simulink model "SLemba_CPG_startup"  (R2024a)
settings: Solver=ode113  StartTime=0.0  StopTime=10  MaxStep=1e-3  RelTol=1e-5  AbsTol=1e-5
InitFcn:
  | parameters;
  | initBusObjects;
  | loadCPGParam_startup;
values from neighbouring files (symbols this model uses):
  kx_sol = out.kx(1)    [loadCPGParam_startup.m]
  tst_sol = out.tst(1)    [loadCPGParam_startup.m]
  tsw_sol = out.tsw(1)    [loadCPGParam_startup.m]
  y_sol = out.q(2,1)    [loadCPGParam_startup.m]
undefined symbols (not defined in the file or in its folder): Init
settings Model: Creator=heath  LastModifiedBy=Mechatronics
settings SolverCC: ZeroCrossControl=EnableAll
settings DebuggingCC: AlgebraicLoopMsg=none

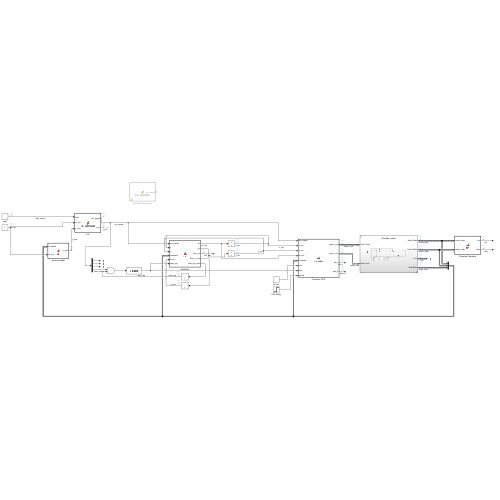
[thumbnail: Simulink's stored preview of the top-level diagram]
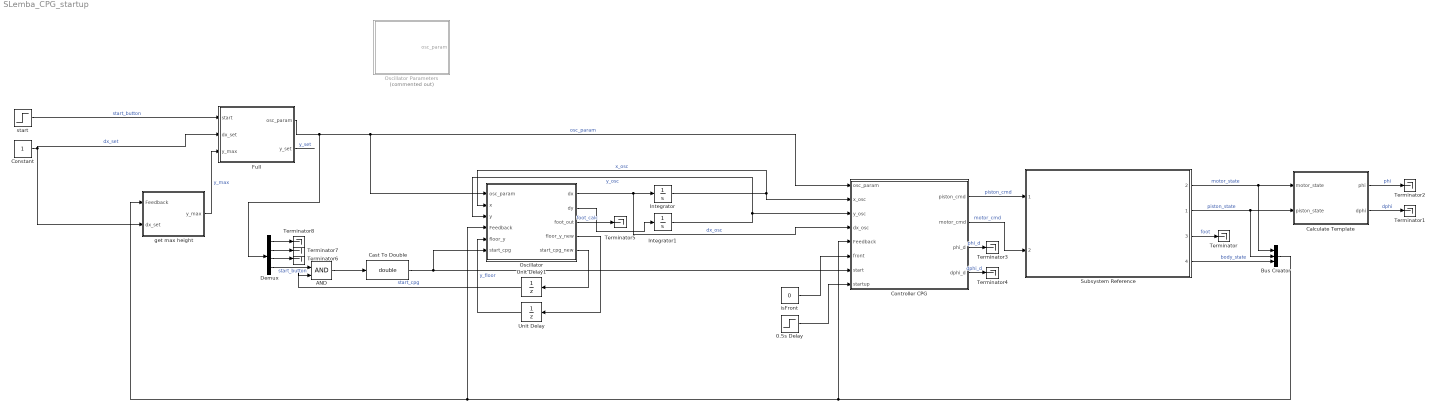
== system SLemba_CPG_startup ==
  0.5s Delay : Step  Time=0.001  SampleTime=0
  AND : Logic  IconShape=distinctive  AllPortsSameDT=off  OutDataTypeStr=boolean
  Bus Creator : BusCreator  Inputs=3  OutDataTypeStr=Bus: State
      settings: InheritFromInputs=off
  Calculate Template : MATLAB Function  TreatAsAtomicUnit=on
  Cast To Double : DataTypeConversion  OutDataTypeStr=double  SaturateOnIntegerOverflow=off  RndMeth=Floor
  Constant : Constant
  Controller CPG : MATLAB Function  TreatAsAtomicUnit=on
  Demux : Demux
  Full : MATLAB Function  TreatAsAtomicUnit=on
  Integrator : Integrator  InitialCondition=Init.CPG(1)
  Integrator1 : Integrator  InitialCondition=Init.CPG(2)
  Oscillator : MATLAB Function  TreatAsAtomicUnit=on
  Oscillator Parameters : MATLAB Function  Commented=on  TreatAsAtomicUnit=on
  Subsystem Reference : Subsystem  ReferencedSubsystem=SLemba_model
      settings: PortSchema="{\"entries\":[{\"content\":{\"sides\":[{\"content\":{\"connectorIds\":[\"In1\",\"In2\"]},\"type\":\"ConnectorPlacement.EquallySpacedRectSide\",\"uuid\":\"d72a35c2-6749-4eaa-8584-fa64d0dc3e1c\"},{\"content\":{\"connectorIds\":[\"Out2\",\"Out1\",\"Out3\",\"Out4\"],\"side\":\"RIGHT\"},\"type\":\"ConnectorPlacement.EquallySpacedRectSide\",\"uuid\":\"d76b7912-ed10-4044-b6e4-c8872f57f584\"},{\"content\":{\"side\":\"TOP\"},\"type\":\"ConnectorPlacement.EquallySpacedRectSide\",\"uuid\":\"b81d1af6-43ba-45da-aadf-2679a7ef4974\"}]},\"type\":\"ConnectorPlacement.EquallySpacedConnector\",\"uuid\":\"64dd74d6-47ac-4ba4-b7a1-dc32513bde35\"}],\"packageUris\":[\"http://schema.mathworks.com/mf0/Connector/R2020b\"],\"version\":\"1.0\"}"
  Terminator{,1..8} (9 alike) : Terminator
  Unit Delay : UnitDelay  SampleTime=-1  HasFrameUpgradeWarning=on
  Unit Delay1 : UnitDelay  SampleTime=-1  HasFrameUpgradeWarning=on
  get max height : MATLAB Function  TreatAsAtomicUnit=on
  isFront : Constant  Value=0
  start : Step  Time=0.002  SampleTime=0
  wires:
  isFront/1 -> Controller CPG/6(front)
  Controller CPG/1(piston_cmd) -> Subsystem Reference/1  "piston_cmd"
  Controller CPG/2(motor_cmd) -> Subsystem Reference/2  "motor_cmd"
  Subsystem Reference/3 -> Terminator/1  "foot"
  Controller CPG/3(phi_d) -> Terminator3/1  "phi_d"
  Controller CPG/4(dphi_d) -> Terminator4/1  "dphi_d"
  Calculate Template/1(phi) -> Terminator2/1  "phi"
  Calculate Template/2(dphi) -> Terminator1/1  "dphi"
  Oscillator/1(dx) -> Controller CPG/4(dx_osc), Integrator/1  "dx_osc"
  Oscillator/2(dy) -> Integrator1/1
  Oscillator/4(floor_y_new) -> Unit Delay/1
  Unit Delay/1 -> Oscillator/5(floor_y)  "y_floor"
  Oscillator/3(foot_out) -> Terminator5/1  "foot_calc"
  start/1 -> Full/1(start)  "start_button"
  Oscillator/5(start_cpg_new) -> Unit Delay1/1
  Subsystem Reference/2 -> Bus Creator/1, Calculate Template/1(motor_state)  "motor_state"
  Subsystem Reference/1 -> Calculate Template/2(piston_state), Bus Creator/2  "piston_state"
  Subsystem Reference/4 -> Bus Creator/3  "body_state"
  Bus Creator/1 -> Controller CPG/5(Feedback), get max height/1(Feedback), Oscillator/4(Feedback)
  0.5s Delay/1 -> Controller CPG/8(startup)
  Constant/1 -> get max height/2(dx_set), Full/2(dx_set)  "dx_set"
  Full/1(osc_param) -> Demux/1, Oscillator/1(osc_param), Controller CPG/1(osc_param)  "osc_param"
  Unit Delay1/1 -> AND/2  "start_cpg"
  Demux/1 -> Terminator8/1
  Demux/2 -> Terminator7/1
  Demux/3 -> Terminator6/1
  Demux/4 -> AND/1  "start_button"
  AND/1 -> Cast To Double/1
  Cast To Double/1 -> Controller CPG/7(start), Oscillator/6(start_cpg)
  get max height/1(y_max) -> Full/3(y_max)  "y_max"
  Full/2(y_set) -> ?  "y_set"
  Integrator/1 -> Controller CPG/2(x_osc), Oscillator/2(x)  "x_osc"
  Integrator1/1 -> Oscillator/3(y), Controller CPG/3(y_osc)  "y_osc"

== matlab function SLemba_CPG_startup/Controller CPG ==
  settings: updateMethod=DISCRETE
  data: osc_param input; x_osc input; piston_cmd output Bus: PistonCmd; y_osc input; dx_osc input; Feedback input Bus: State; front input; start input; startup input double; motor_cmd output Bus: MotorCmd; phi_d output; dphi_d output
function [piston_cmd,motor_cmd,phi_d,dphi_d] = Controller(osc_param, x_osc,y_osc,dx_osc,Feedback,front, start, startup)

persistent state_control % 1 = wait, 2 = startup, 3 = stop

if isempty(state_control)
    state_control = 1;
end


motor_state = Feedback.Motor; piston_state = Feedback.Piston;

kx = osc_param(3);

l = piston_state.p;
dl = piston_state.v;
th = motor_state.q;

if (front)
    direction = -1;
else
    direction = 1;
end

% set command
phi_d = direction*x_osc*kx + pi/2;
dphi_d = direction*dx_osc*kx;
if (y_osc>0) 
    if(x_osc>0)
        ue = 0; ur = 1;
    else
            ue = 1; ur = 1;
    end
else
    ue = 1; ur = 0;
end

kp = 250;
kd = 10;

% % Testing
% % ----------
% ue = 1; ur = 0;
% phi_d = pi/2; dphi_d = 0;
% kp = 250;kd = 5;
% % ---------

if start == 0
    ue = 0; ur = 1;
    phi_d = pi/2; dphi_d = 0;
end

switch(state_control)
    case 1
        if startup == 1
            state_control = 2;
        end
end

switch(state_control)
    case 2
        piston_cmd.ue = ue;
        piston_cmd.ur = ur;
        
        motor_cmd.q = th_calc(phi_d,l);
        motor_cmd.w = dth_calc(phi_calc(th,l),l,dphi_d,dl);
        motor_cmd.Kp = kp;
        motor_cmd.Kd = kd;
        motor_cmd.tff = 0;
    otherwise
        piston_cmd.ue = 0;
        piston_cmd.ur = 0;
        
        motor_cmd.q = 0;
        motor_cmd.w = 0;
        motor_cmd.Kp = 0;
        motor_cmd.Kd = 0;
        motor_cmd.tff = 0;
end

== matlab function SLemba_CPG_startup/Oscillator ==
  settings: updateMethod=DISCRETE
  data: osc_param input; x input size=1; dx output size=1; y input; Feedback input; dy output; foot_out output; floor_y_new output; floor_y input; start_cpg input; start_cpg_new output
function [dx,dy,foot_out,floor_y_new,start_cpg_new] = CPG(osc_param,x,y,Feedback, floor_y, start_cpg)%,dy_lift, fit)%dq_osc = CPG(input_osc)%
% x = input_osc.x_osc; y = input_osc.y_osc; osc_param = input_osc.osc_param;
% Body_state = input_osc.Body_state; Piston_state = input_osc.Piston_state; Motor_state = input_osc.Motor_state;

persistent thrown

if isempty(thrown)
    thrown = 0;
end

Body_state = Feedback.Body; Motor_state = Feedback.Motor; Piston_state = Feedback.Piston;

x_body = Body_state.x; y_body = Body_state.y;
dx_body = Body_state.dx; dy_body = Body_state.dy;
th = Motor_state.q; dth = Motor_state.w;
l = Piston_state.p; dl = Piston_state.v;

thk = thk_calc(th,l); tha = tha_calc(th,l);
dthk = dthk_calc(th,l,dth,dl); dtha = dtha_calc(th,l,dth,dl);

foot = foot_Func(x_body,y_body,th,l,thk,tha,dx_body,dy_body,dth,dl,dthk,dtha);

y_foot = foot(2);
dy_foot = foot(4);

% update floor height based on accelerometer impact
% only activates if system is running and osc is in correct quadrant
ddy_tol = 30;
if (Body_state.ddy > ddy_tol && osc_param(4) && x<-0.5)
    floor_y = y_foot;
end

% start cpg if in correct state once thrown
dy_tol = 0.2;

if dy_body>dy_tol && osc_param(4)
    thrown = 1;
end

if(thrown && dy_body<0)
% if(osc_param(4))
    start_cpg_new = 1;
else
    start_cpg_new = start_cpg;
end

y_foot = y_foot - floor_y;

foot(2) = y_foot;
foot_out = foot;

floor_y_new = floor_y;

tst = osc_param(1);
tsw = osc_param(2);

% constants
mu = 1;
F_1 = 50;
gamma = 10;
b = 100;


% if(dy_lift>0)
%     coeff = fit.coeff;
% 
%     tsw_new = coeff(1) + coeff(2)*tst + coeff(3)*dy_lift + coeff(4)*tst^2 + coeff(5)*tst*dy_lift + coeff(6)*dy_lift^2;
%     if (tsw_new>tst)
%         tsw = tsw_new;
%     end
% end


T = tst + tsw;
d = tsw/T;
% 
% % 3 frequencies with quadrant crossover
% omega_1 = pi/(T*d);
% omega_2 = omega_1;
% omega_3 = pi/(T - T*d);

k = 1; % 2 for extension at half way
e = 0;%0.4;

% 3 frequencies with quadrant crossover
omega_1 = (pi*k - 2*d*e + 2*d*e*k + pi)/(2*T*d*k);
omega_2 = k*omega_1;
omega_3 = (pi*k - 2*d*e + 2*d*e*k + pi)/(T - T*d + T*k - T*d*k);

% polar coordinates
r = sqrt(x^2 + y^2);
th = atan2(y,x);
% th = atan(y/x);
% if (x <= 0)
%     th = pi + atan(y/x);
% end

% 3 frequencies with quadrant cross over
k1 = omega_1/((exp(-b*(x))+1)*(exp(-b*y)+1));
k2 = omega_2/((exp(b*(x))+1)*(exp(-b*y)+1));
k3 = omega_3/(exp(b*y)+1);
omega = k1 + k2 + k3;

f = @(v) 1 + 0.5*cos(v)*tanh(sin(2*v));
f_dash = @(v) cos(v)*cos(2*v)*(sech(sin(2*v)))^2-0.5*sin(v)*tanh(sin(2*v));

% oscillation
dth = omega;
dr = mu*omega*f_dash(th) + gamma*(mu*f(th)-r);

% change in x
dx = dr*cos(th) - r*sin(th)*dth;

if (y_foot <= 0 && y > 0 && x < 0) % fast transition case 1
    u = -F_1;
elseif(y_foot > 0 && y < 0 && x > 0) % fast transition case 3
    u = F_1;
elseif (y < 0 && dy_foot < 0 && y_foot > 0) % slow transition case 2
    u = - omega*x;
else
    u = 0;
end

dy = dr*sin(th) + r*cos(th)*dth + u;

if start_cpg == 0
    dy = 0;
    dx = 0;
end
end

== matlab function SLemba_CPG_startup/Oscillator Parameters ==
  data: osc_param output; CPG parameter
function osc_param = osc_paramCalc(CPG)

% persistent osc_paramVal
% 
% if isempty(osc_paramVal)
%     out = load("PSO_runs/sol.mat");
%     out = out.out;
%     tst = out.simParams.tst;
%     kx = out.simParams.kx;
% 
%     tsw = out.out.BestSol.Position(4);
% 
%     osc_paramVal = [tst,tsw,kx];
% end

tst = CPG.tst;
kx = CPG.kx;
tsw = CPG.tsw;

osc_param = [tst,tsw,kx];

== matlab function SLemba_CPG_startup/Calculate Template ==
  data: motor_state input; phi output; piston_state input; dphi output
function [phi,dphi] = fcn(motor_state,piston_state)

phi = phi_calc(motor_state.q,piston_state.p);
dphi = dphi_calc(motor_state.q,piston_state.p,motor_state.w,piston_state.v);

== matlab function SLemba_CPG_startup/Full ==
  data: osc_param output; tst_sol parameter; kx_sol parameter; tsw_sol parameter; start input; dx_set input; y_max input; y_sol parameter; y_set output
function [osc_param,y_set] = osc_paramCalc(tst_sol, kx_sol, tsw_sol,start, dx_set,y_max, y_sol)

% persistent osc_paramVal
% 
% if isempty(osc_paramVal)
%     out = load("PSO_runs/sol.mat");
%     out = out.out;
%     tst = out.simParams.tst;
%     kx = out.simParams.kx;
% 
%     tsw = out.out.BestSol.Position(4);
% 
%     osc_paramVal = [tst,tsw,kx];
% end

k_h = 2;

persistent state % 0 is wait, 1 is green button pressed to start

if isempty(state)
    state = 0;
end

switch(state)
    case 0
        if(start)
            state = 1;
        end
end

tst = 0;
kx = 0;
tsw = 0;
y_set = 0;

if state
    
    y_set = polyval(y_sol,dx_set);

    tst = polyval(tst_sol,dx_set);% + k_h*(y_set - y_max);
    kx = polyval(kx_sol,dx_set);
    tsw = polyval(tsw_sol,dx_set);
end

osc_param = [tst,tsw,kx,state];

== matlab function SLemba_CPG_startup/get max height ==
  settings: updateMethod=DISCRETE
  data: Feedback input; dx_set input; y_max output; y_sol parameter
function y_max = fcn(Feedback,dx_set,y_sol)

Body = Feedback.Body; Piston = Feedback.Piston;

persistent y_maxVal % previous maximum height of hop

if isempty(y_maxVal)
    y_maxVal = polyval(y_sol,dx_set);
end

if (abs(Body.dy)<0.05 && Body.ddy < 0 && Piston.p <= 0)
    y_maxVal = Body.y;
end

y_max = y_maxVal;
